simulink model "Project4_MODEL"  (R2023b)
settings: Solver=VariableStepAuto  StartTime=0.0  StopTime=200  RelTol=1e-3
values from neighbouring files (symbols this model uses):
  xp = [sx1 , R*cos(t1) + L , sx2, R*cos(t2)]    [Project_Final_Code.m]
  yp = [sy1, R*sin(t1) + R-offset , sy2 , R*sin(t2) + R-offset]    [Project_Final_Code.m]
undefined symbols (not defined in the file or in its folder): batData, carData, motorData
libraries: slpidlib x1
settings Model: Creator=saman  LastModifiedBy=saman

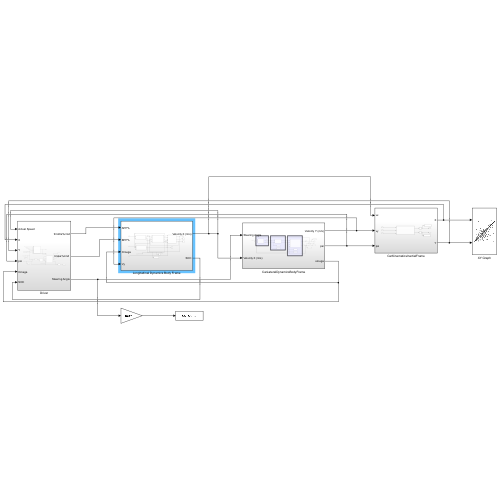
[thumbnail: Simulink's stored preview of the top-level diagram]
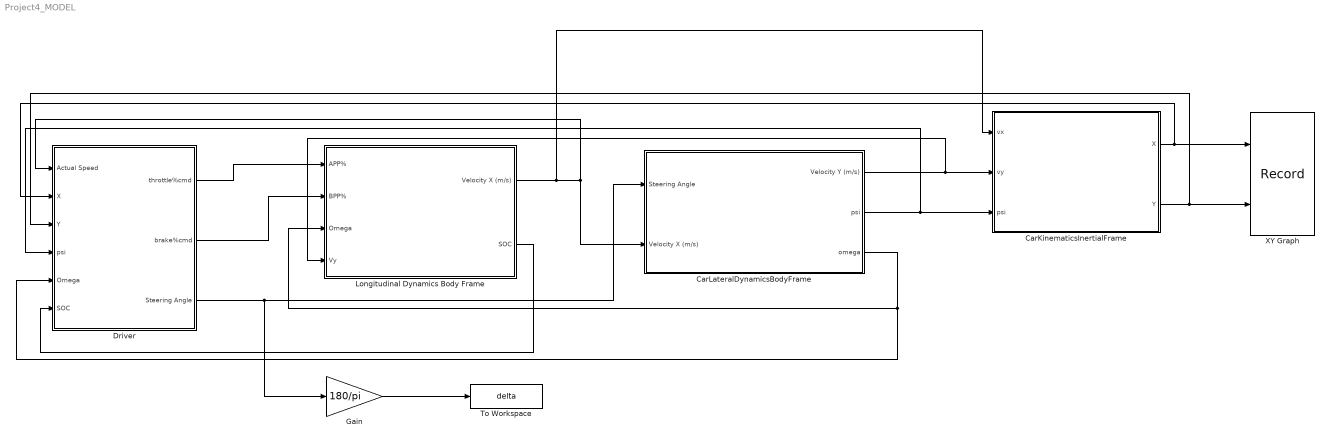
== system Project4_MODEL ==
  CarKinematicsInertialFrame : Subsystem
  CarLateralDynamicsBodyFrame : Subsystem
  "Driver " : Subsystem
  Gain : Gain  Gain=180/pi
  Longitudinal Dynamics Body Frame : Subsystem
  To Workspace : ToWorkspace  VariableName=delta  SaveFormat=Timeseries  SampleTime=-1
  XY Graph : Record  FileSettingsInternal="{\"entries\":[{\"content\":{\"excelSettings\":{\"content\":{},\"type\":\"Streamout.ExcelSettings\"}},\"type\":\"Streamout.FileSettingStorage\",\"uuid\":\"\"}],\"packageUris\":[\"http:\\/\\/schema.mathworks.com\\/mf0\\/streamout_blocks\\/R2020a\"],\"version\":\"1.0\"}"  Layout=[1 1]  SignalsInternal="{\"entries\":[{\"content\":{\"signals\":[{\"content\":{\"blockPath\":[],\"dimensions\":[1],\"domain\":\"\",\"lineColor\":\"#a2142f\",\"plots\":[1],\"port\":1,\"sid\":[\"\"],\"signalID\":55552,\"signalName\":\"CarKinematicsInertialFrame:1\"},\"type\":\"RecordBlkView.Signal\",\"uuid\":\"\"},{\"content\":{\"blockPath\":[],\"dimensions\":[1],\"domain\":\"\",\"lineColor\":\"#139fff\",\"plots\":[1],\"port\":2,\"sid\":[\"\"],\"signalID\":55556,\"signalName\":\"CarKinematicsInertialFrame:2\"},\"type\":\"RecordBlkView.Signal\",\"uuid\":\"\"}]},\"type\":\"RecordBlkView.InputSignals\",\"uuid\":\"\"}],\"packageUris\":[\"http:\\/\\/schema.mathworks.com\\/mf0\\/streamout_blocks\\/R2020a\"],\"version\":\"1.0\"}"  VisualizationBindings="{\"xyplotplugin\":{\"info\":[{\"series\":[{\"bindingParametersList\":[{\"parameter\":\"X-Axis\",\"signalID\":55552,\"signalName\":\"CarKinematicsInertialFrame:1\"},{\"parameter\":\"Y-Axis\",\"signalID\":55556,\"signalName\":\"CarKinematicsInertialFrame:2\"}],\"seriesID\":61892}],\"subplotID\":1}]}}"  CompatibilityTag=XY  st=-1
  wires:
  CarLateralDynamicsBodyFrame/2(psi) -> "Driver "/4(psi), CarKinematicsInertialFrame/3(psi)
  CarKinematicsInertialFrame/2(Y) -> "Driver "/3(Y), XY Graph/2
  CarKinematicsInertialFrame/1(X) -> XY Graph/1, "Driver "/2(X)
  CarLateralDynamicsBodyFrame/1(Velocity Y (m/s)) -> Longitudinal Dynamics Body Frame/4(Vy), CarKinematicsInertialFrame/2(vy)
  "Driver "/1(throttle%cmd) -> Longitudinal Dynamics Body Frame/1(APP%)
  "Driver "/2("brake%cmd ") -> Longitudinal Dynamics Body Frame/2(BPP%)
  Longitudinal Dynamics Body Frame/1(Velocity X (m/s)) -> CarKinematicsInertialFrame/1(vx), "Driver "/1(Actual Speed), CarLateralDynamicsBodyFrame/2(Velocity X (m/s))
  Longitudinal Dynamics Body Frame/2(SOC) -> "Driver "/6(SOC)
  CarLateralDynamicsBodyFrame/3(omega) -> Longitudinal Dynamics Body Frame/3(Omega), "Driver "/5(Omega)
  "Driver "/3(Steering Angle) -> Gain/1, CarLateralDynamicsBodyFrame/1(Steering Angle)
  Gain/1 -> To Workspace/1

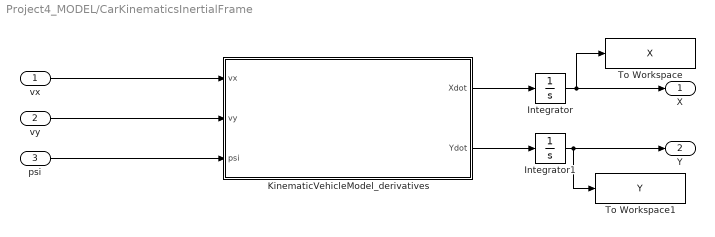
== system Project4_MODEL/CarKinematicsInertialFrame ==
  vx : Inport
  vy : Inport  Port=2
  psi : Inport  Port=3
  Integrator : Integrator  InitialCondition=carData.init.X0
  Integrator1 : Integrator  InitialCondition=carData.init.Y0
  KinematicVehicleModel_derivatives : MATLAB Function  TreatAsAtomicUnit=on  mask{obj=carData}
      mask prompts: obj "obj structure"
  To Workspace : ToWorkspace  VariableName=X  SaveFormat=Timeseries  SampleTime=-1
  To Workspace1 : ToWorkspace  VariableName=Y  SaveFormat=Timeseries  SampleTime=-1
  X : Outport
  Y : Outport  Port=2
  wires:
  KinematicVehicleModel_derivatives/1(Xdot) -> Integrator/1
  KinematicVehicleModel_derivatives/2(Ydot) -> Integrator1/1
  Integrator/1 -> To Workspace/1, X/1
  Integrator1/1 -> To Workspace1/1, Y/1
  vx/1 -> KinematicVehicleModel_derivatives/1(vx)
  vy/1 -> KinematicVehicleModel_derivatives/2(vy)
  psi/1 -> KinematicVehicleModel_derivatives/3(psi)

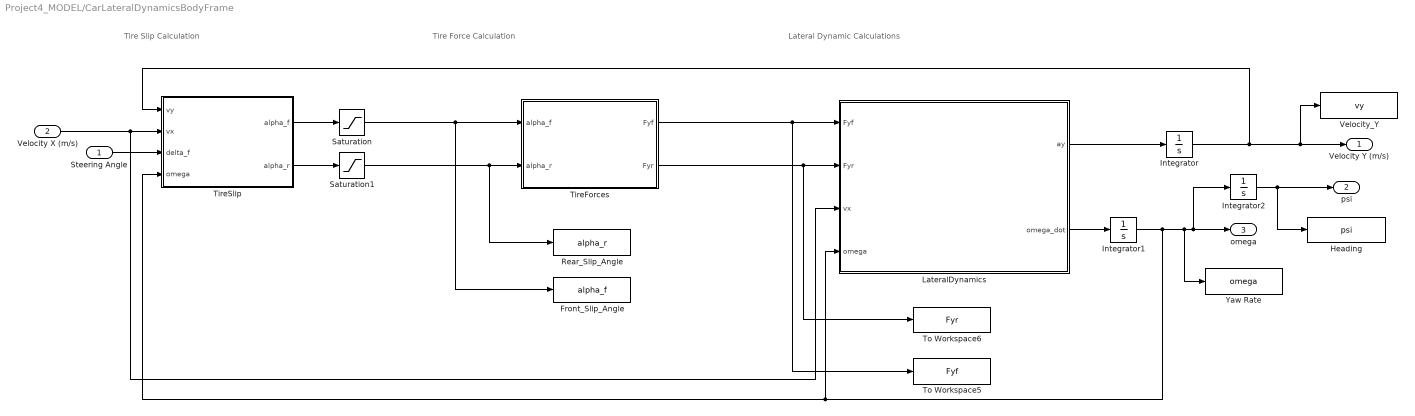
== system Project4_MODEL/CarLateralDynamicsBodyFrame ==
  note: Tire Slip Calculation
  note: Tire Force Calculation
  note: Lateral Dynamic Calculations
  Steering Angle : Inport
  Velocity X (m/s) : Inport  Port=2
  Front_Slip_Angle : ToWorkspace  VariableName=alpha_f  SaveFormat=Timeseries  SampleTime=-1
  Heading : ToWorkspace  VariableName=psi  SaveFormat=Timeseries  SampleTime=-1
  Integrator : Integrator  InitialCondition=carData.init.vy0
  Integrator1 : Integrator  InitialCondition=carData.init.omega0
  Integrator2 : Integrator  InitialCondition=carData.init.psi0
  LateralDynamics : MATLAB Function  TreatAsAtomicUnit=on  mask{obj=carData}
      mask prompts: obj "obj structure"
  Rear_Slip_Angle : ToWorkspace  VariableName=alpha_r  SaveFormat=Timeseries  SampleTime=-1
  Saturation : Saturate  UpperLimit=carData.maxAlpha  LowerLimit=-carData.maxAlpha
  Saturation1 : Saturate  UpperLimit=carData.maxAlpha  LowerLimit=-carData.maxAlpha
  TireForces : MATLAB Function  TreatAsAtomicUnit=on  mask{obj=carData}
      mask prompts: obj "obj structure"
  TireSlip : MATLAB Function  TreatAsAtomicUnit=on  mask{obj=carData}
      mask prompts: obj "obj structure"
  To Workspace5 : ToWorkspace  VariableName=Fyf  SaveFormat=Timeseries  SampleTime=-1
  To Workspace6 : ToWorkspace  VariableName=Fyr  SaveFormat=Timeseries  SampleTime=-1
  Velocity_Y : ToWorkspace  VariableName=vy  SaveFormat=Timeseries  SampleTime=-1
  Yaw Rate : ToWorkspace  VariableName=omega  SaveFormat=Timeseries  SampleTime=-1
  Velocity Y (m/s) : Outport
  psi : Outport  Port=2
  omega : Outport  Port=3
  wires:
  LateralDynamics/1(ay) -> Integrator/1
  Integrator/1 -> Velocity Y (m/s)/1, Velocity_Y/1, TireSlip/1(vy)
  LateralDynamics/2(omega_dot) -> Integrator1/1
  Integrator1/1 -> Integrator2/1, omega/1, Yaw Rate/1, LateralDynamics/4(omega), TireSlip/4(omega)
  TireSlip/1(alpha_f) -> Saturation/1
  TireSlip/2(alpha_r) -> Saturation1/1
  TireForces/1(Fyf) -> LateralDynamics/1(Fyf), To Workspace5/1
  TireForces/2(Fyr) -> LateralDynamics/2(Fyr), To Workspace6/1
  Saturation/1 -> TireForces/1(alpha_f), Front_Slip_Angle/1
  Saturation1/1 -> TireForces/2(alpha_r), Rear_Slip_Angle/1
  Velocity X (m/s)/1 -> TireSlip/2(vx), LateralDynamics/3(vx)
  Steering Angle/1 -> TireSlip/3(delta_f)
  Integrator2/1 -> Heading/1, psi/1

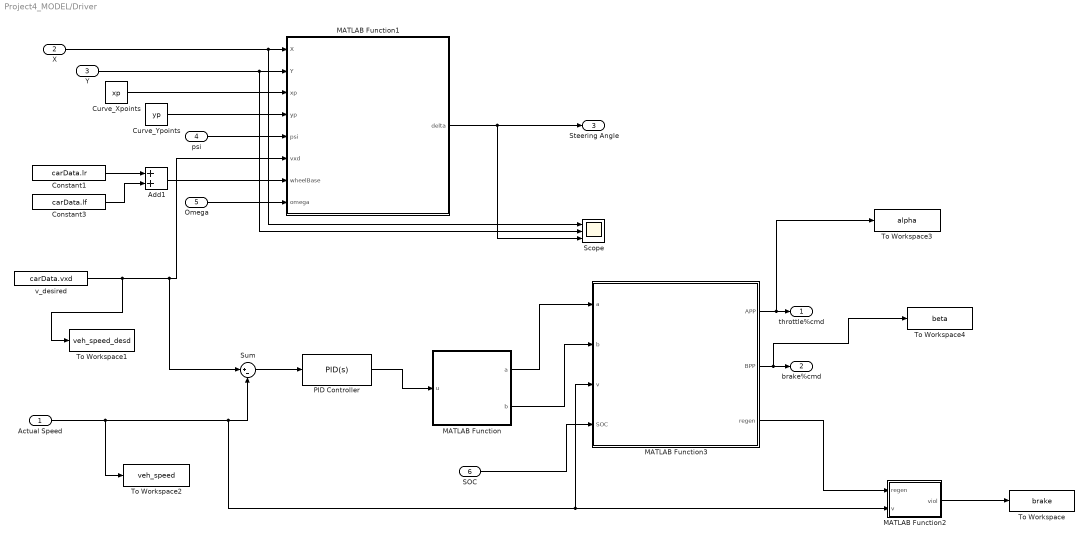
== system Project4_MODEL/Driver  ==
  Actual Speed : Inport
  X : Inport  Port=2
  Y : Inport  Port=3
  psi : Inport  Port=4
  Omega : Inport  Port=5
  SOC : Inport  Port=6
  Add1 : Sum
  Constant1 : Constant  Value=carData.lr
  Constant3 : Constant  Value=carData.lf
  Curve_Xpoints : Constant  Value=xp  VectorParams1D=off
  Curve_Ypoints : Constant  Value=yp  VectorParams1D=off
  MATLAB Function : MATLAB Function  TreatAsAtomicUnit=on
  MATLAB Function1 : MATLAB Function  TreatAsAtomicUnit=on
  MATLAB Function2 : MATLAB Function  TreatAsAtomicUnit=on
  MATLAB Function3 : MATLAB Function  TreatAsAtomicUnit=on
  PID Controller : slpidlib/PID Controller  Controller=PID  Form=Parallel  TimeDomain=Continuous-time  UseExternalTs=off  SampleTime=-1  IntegratorMethod=Forward Euler  FilterMethod=Forward Euler  ControllerParametersSource=internal  P=2.5  I=.1  UseKiTs=off  D=.5  N=100  UseFilter=on  TunerSelectOption=Transfer Function Based (PID Tuner App)  InitialConditionSource=internal  InitialConditionForIntegrator=0  InitialConditionForFilter=0  DifferentiatorICPrevScaledInput=0  ExternalReset=none  TrackingMode=off  Kt=1  LimitOutput=on  SatLimitsSource=internal  UpperSaturationLimit=1  LowerSaturationLimit=-1  LinearizeAsGain=off  AntiWindupMode=none  Kb=1  LimitIntegrator=off  UpperIntegratorSaturationLimit=inf  LowerIntegratorSaturationLimit=-inf  POutMin=[]  POutMax=[]  IOutMin=[]  IOutMax=[]  DOutMin=[]  DOutMax=[]  NOutMin=[]  NOutMax=[]  SumOutMin=[]  SumOutMax=[]  SaturationOutMin=[]  SaturationOutMax=[]  PParamMin=[]  PParamMax=[]  IParamMin=[]  IParamMax=[]  DParamMin=[]  DParamMax=[]  NParamMin=[]  NParamMax=[]  KbParamMin=[]  KbParamMax=[]  KtParamMin=[]  KtParamMax=[]  KbOutMin=[]  KbOutMax=[]  KtOutMin=[]  KtOutMax=[]  IntegratorOutMin=[]  IntegratorOutMax=[]  FilterOutMin=[]  FilterOutMax=[]  SumI1OutMin=[]  SumI1OutMax=[]  SumI2OutMin=[]  SumI2OutMax=[]  SumI3OutMin=[]  SumI3OutMax=[]  SumI4OutMin=[]  SumI4OutMax=[]  SumDOutMin=[]  SumDOutMax=[]  DifferentiatorOutMin=[]  DifferentiatorOutMax=[]  FilterDiffOutCoefMin=[]  FilterDiffOutCoefMax=[]  ReciprocalOutMin=[]  ReciprocalOutMax=[]  SumDenOutMin=[]  SumDenOutMax=[]  SumNumOutMin=[]  SumNumOutMax=[]  DivideOutMin=[]  DivideOutMax=[]  UdiffTsProdOutMin=[]  UdiffTsProdOutMax=[]  NTsProdOutMin=[]  NTsProdOutMax=[]  UintegralTsProdOutMin=[]  UintegralTsProdOutMax=[]  UngainTsProdOutMin=[]  UngainTsProdOutMax=[]  ClampingZeroOutDataTypeStr=Inherit: Inherit via back propagation  ClampingZeroOutMin=[]  ClampingZeroOutMax=[]  FilterDenConstantOutDataTypeStr=Inherit: Inherit via back propagation  FilterDenConstantOutMin=[]  FilterDenConstantOutMax=[]  PCopyOutDataTypeStr=Inherit: Inherit via back propagation  PCopyOutMin=[]  PCopyOutMax=[]  NCopyOutDataTypeStr=Inherit: Inherit via back propagation  NCopyOutMin=[]  NCopyOutMax=[]  IntegratorContinuousStateAttributes=''  IntegratorStateMustResolveToSignalObject=off  IntegratorRTWStateStorageClass=Auto  FilterContinuousStateAttributes=''  FilterStateMustResolveToSignalObject=off  FilterRTWStateStorageClass=Auto  ParallelPVariant=InternalParameters  IdealPVariant=Disabled  IVariant=InternalParameters  DVariant=InternalParameters  IntegratorVariant=Continuous  SatVariant=Enabled  AWVariant=Passthrough  PCopyVariant=Disabled  TRVariant=Disabled  FdbkBlocksVariant=Forward  IdealPFdbkVariant=Disabled  SatFdbkVariant=Disabled  DerivativeFilterVariant=ContFilter  NVariant=InternalParameters  NCopyVariant=Disabled  FilterICVariant=InternalICsFilter  IntegratorICVariant=InternalICs  ExternalResetVariant=Disabled  TRSumVariant=Passthrough  SumFdbkVariant=Disabled  SumVariant=Sum_PID  TsampFilterVariant=InternalTs  TsampNgainVariant=Passthrough  TsampIntegralVariant=Disabled_SignalSpec  ExternalSaturationOutDataTypeStr=Inherit: Same as second input
  Scope : Scope  NumInputPorts=3
  Sum : Sum  Inputs=|+-
  To Workspace : ToWorkspace  VariableName=brake  SaveFormat=Timeseries  SampleTime=-1
  To Workspace1 : ToWorkspace  VariableName=veh_speed_desd  SaveFormat=Timeseries  SampleTime=-1
  To Workspace2 : ToWorkspace  VariableName=veh_speed  SaveFormat=Timeseries  SampleTime=-1
  To Workspace3 : ToWorkspace  VariableName=alpha  SaveFormat=Timeseries  SampleTime=-1
  To Workspace4 : ToWorkspace  VariableName=beta  SaveFormat=Timeseries  SampleTime=-1
  v_desired : Constant  Value=carData.vxd
  throttle%cmd : Outport
  "brake%cmd " : Outport  Port=2
  Steering Angle : Outport  Port=3
  wires:
  v_desired/1 -> To Workspace1/1, Sum/1, MATLAB Function1/6(vxd)
  Actual Speed/1 -> To Workspace2/1, MATLAB Function3/3(v), MATLAB Function2/2(v), Sum/2
  Sum/1 -> PID Controller/1
  PID Controller/1 -> MATLAB Function/1(u)
  Omega/1 -> MATLAB Function1/8(omega)
  Curve_Ypoints/1 -> MATLAB Function1/4(yp)
  psi/1 -> MATLAB Function1/5(psi)
  X/1 -> Scope/1, MATLAB Function1/1(X)
  Curve_Xpoints/1 -> MATLAB Function1/3(xp)
  MATLAB Function1/1(delta) -> Steering Angle/1, Scope/3
  Y/1 -> Scope/2, MATLAB Function1/2(Y)
  Constant3/1 -> Add1/2
  Constant1/1 -> Add1/1
  Add1/1 -> MATLAB Function1/7(wheelBase)
  MATLAB Function/1(a) -> MATLAB Function3/1(a)
  MATLAB Function/2(b) -> MATLAB Function3/2(b)
  MATLAB Function2/1(viol) -> To Workspace/1
  SOC/1 -> MATLAB Function3/4(SOC)
  MATLAB Function3/3(regen) -> MATLAB Function2/1(regen)
  MATLAB Function3/2(BPP) -> To Workspace4/1, "brake%cmd "/1
  MATLAB Function3/1(APP) -> To Workspace3/1, throttle%cmd/1

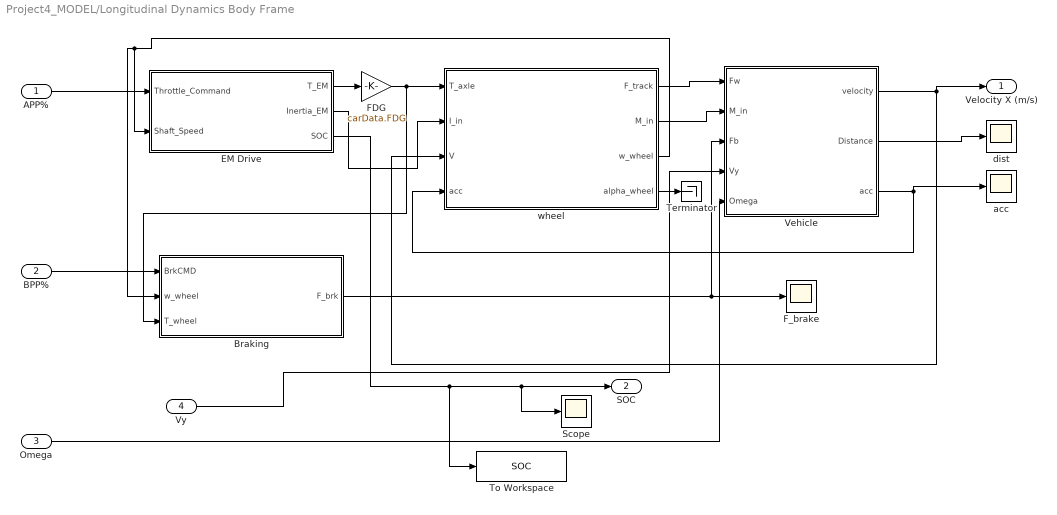
== system Project4_MODEL/Longitudinal Dynamics Body Frame ==
  APP% : Inport
  BPP% : Inport  Port=2
  Omega : Inport  Port=3
  Vy : Inport  Port=4
  Braking : Subsystem
  EM Drive : Subsystem
  FDG : Gain  Gain=carData.FDG
  F_brake : Scope
  Scope : Scope
  Terminator : Terminator
  To Workspace : ToWorkspace  VariableName=SOC  SaveFormat=Timeseries  SampleTime=-1
  Vehicle : Subsystem
  acc : Scope
  dist : Scope
  "wheel " : Subsystem
  Velocity X (m/s) : Outport
  SOC : Outport  Port=2
  wires:
  "wheel "/3(w_wheel) -> Braking/2("w_wheel "), EM Drive/2(Shaft_Speed)
  Vehicle/3(acc) -> acc/1, "wheel "/4(acc)
  Braking/1("F_brk ") -> Vehicle/3("Fb "), F_brake/1
  "wheel "/2(M_in) -> Vehicle/2("M_in ")
  Vehicle/1("velocity ") -> Velocity X (m/s)/1, "wheel "/3(V)
  "wheel "/1(F_track) -> Vehicle/1("Fw ")
  EM Drive/3(SOC) -> To Workspace/1, Scope/1, SOC/1
  FDG/1 -> Braking/3(T_wheel), "wheel "/1(T_axle)
  EM Drive/2(Inertia_EM) -> "wheel "/2(I_in)
  Vehicle/2("Distance ") -> dist/1
  "wheel "/4(alpha_wheel) -> Terminator/1
  EM Drive/1(T_EM) -> FDG/1
  APP%/1 -> EM Drive/1(Throttle_Command)
  BPP%/1 -> Braking/1("BrkCMD ")
  Vy/1 -> Vehicle/4(Vy)
  Omega/1 -> Vehicle/5(Omega)

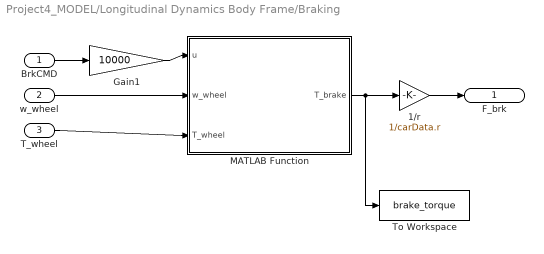
== system Project4_MODEL/Longitudinal Dynamics Body Frame/Braking ==
  "BrkCMD " : Inport
  "w_wheel " : Inport  Port=2
  T_wheel : Inport  Port=3
  1/r : Gain  Gain=1/carData.r
  Gain1 : Gain  Gain=10000
  MATLAB Function : MATLAB Function  TreatAsAtomicUnit=on
  To Workspace : ToWorkspace  VariableName=brake_torque  SaveFormat=Timeseries  SampleTime=-1
  "F_brk " : Outport  VectorParamsAs1DForOutWhenUnconnected=off
  wires:
  "BrkCMD "/1 -> Gain1/1
  Gain1/1 -> MATLAB Function/1(u)
  MATLAB Function/1(T_brake) -> To Workspace/1, 1/r/1
  "w_wheel "/1 -> MATLAB Function/2(w_wheel)
  T_wheel/1 -> MATLAB Function/3(T_wheel)
  1/r/1 -> "F_brk "/1

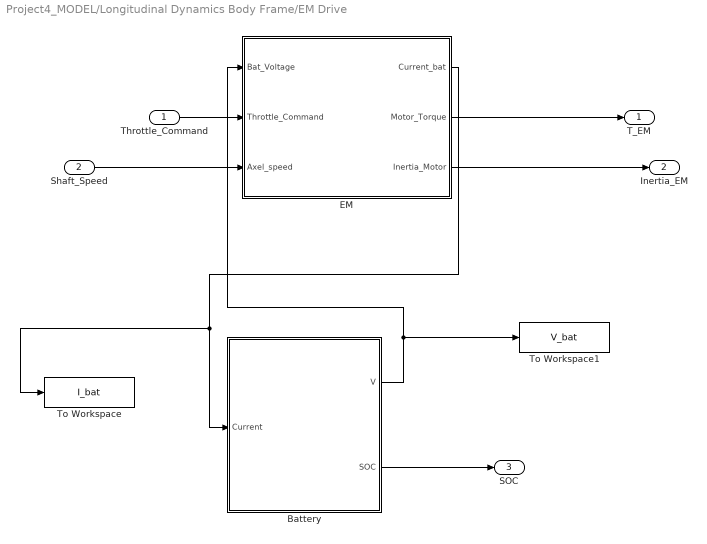
== system Project4_MODEL/Longitudinal Dynamics Body Frame/EM Drive ==
  Throttle_Command : Inport
  Shaft_Speed : Inport  Port=2
  Battery : Subsystem
  EM : Subsystem
  To Workspace : ToWorkspace  VariableName=I_bat  SaveFormat=Timeseries  SampleTime=-1
  To Workspace1 : ToWorkspace  VariableName=V_bat  SaveFormat=Timeseries  SampleTime=-1
  T_EM : Outport
  Inertia_EM : Outport  Port=2
  SOC : Outport  Port=3
  wires:
  EM/1(Current_bat) -> To Workspace/1, Battery/1(Current)
  Throttle_Command/1 -> EM/2(Throttle_Command)
  Shaft_Speed/1 -> EM/3(Axel_speed)
  EM/2(Motor_Torque) -> T_EM/1
  EM/3(Inertia_Motor) -> Inertia_EM/1
  Battery/1(V) -> To Workspace1/1, EM/1(Bat_Voltage)
  Battery/2(SOC) -> SOC/1

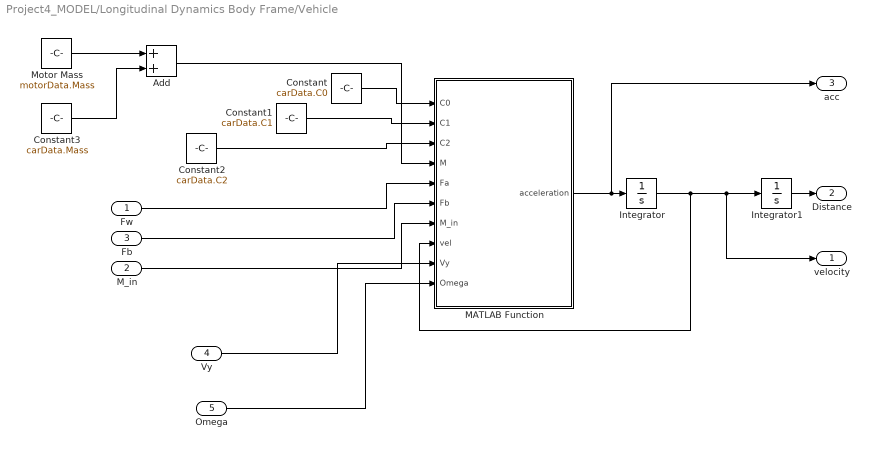
== system Project4_MODEL/Longitudinal Dynamics Body Frame/Vehicle ==
  "Fw " : Inport
  "M_in " : Inport  Port=2
  "Fb " : Inport  Port=3
  Vy : Inport  Port=4
  Omega : Inport  Port=5
  Add : Sum
  Constant : Constant  Value=carData.C0
  Constant1 : Constant  Value=carData.C1
  Constant2 : Constant  Value=carData.C2
  Constant3 : Constant  Value=carData.Mass
  Integrator : Integrator  LimitOutput=on  LowerSaturationLimit=0
  Integrator1 : Integrator
  MATLAB Function : MATLAB Function  TreatAsAtomicUnit=on
  Motor Mass : Constant  Value=motorData.Mass
  "velocity " : Outport  VectorParamsAs1DForOutWhenUnconnected=off
  "Distance " : Outport  Port=2  VectorParamsAs1DForOutWhenUnconnected=off
  acc : Outport  Port=3
  wires:
  Constant1/1 -> MATLAB Function/2(C1)
  Constant/1 -> MATLAB Function/1(C0)
  MATLAB Function/1(acceleration) -> acc/1, Integrator/1
  Constant2/1 -> MATLAB Function/3(C2)
  Constant3/1 -> Add/2
  "Fw "/1 -> MATLAB Function/5(Fa)
  "Fb "/1 -> MATLAB Function/6(Fb)
  Integrator/1 -> MATLAB Function/8(vel), "velocity "/1, Integrator1/1
  Integrator1/1 -> "Distance "/1
  "M_in "/1 -> MATLAB Function/7(M_in)
  Motor Mass/1 -> Add/1
  Add/1 -> MATLAB Function/4(M)
  Vy/1 -> MATLAB Function/9(Vy)
  Omega/1 -> MATLAB Function/10(Omega)

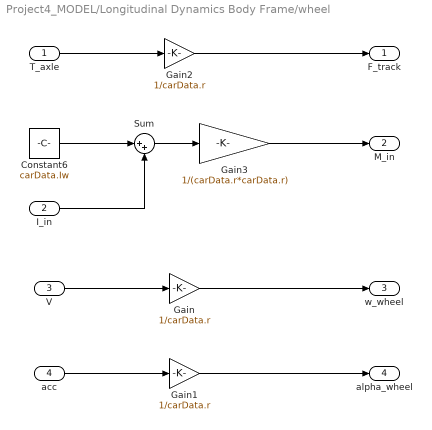
== system Project4_MODEL/Longitudinal Dynamics Body Frame/wheel  ==
  T_axle : Inport
  I_in : Inport  Port=2
  V : Inport  Port=3
  acc : Inport  Port=4
  Constant6 : Constant  Value=carData.Iw
  Gain : Gain  Gain=1/carData.r
  Gain1 : Gain  Gain=1/carData.r
  Gain2 : Gain  Gain=1/carData.r
  Gain3 : Gain  Gain=1/(carData.r*carData.r)
  Sum : Sum  Inputs=|++
  F_track : Outport
  M_in : Outport  Port=2
  w_wheel : Outport  Port=3
  alpha_wheel : Outport  Port=4
  wires:
  Gain/1 -> w_wheel/1
  V/1 -> Gain/1
  acc/1 -> Gain1/1
  Gain1/1 -> alpha_wheel/1
  T_axle/1 -> Gain2/1
  Gain2/1 -> F_track/1
  Gain3/1 -> M_in/1
  Constant6/1 -> Sum/1
  I_in/1 -> Sum/2
  Sum/1 -> Gain3/1

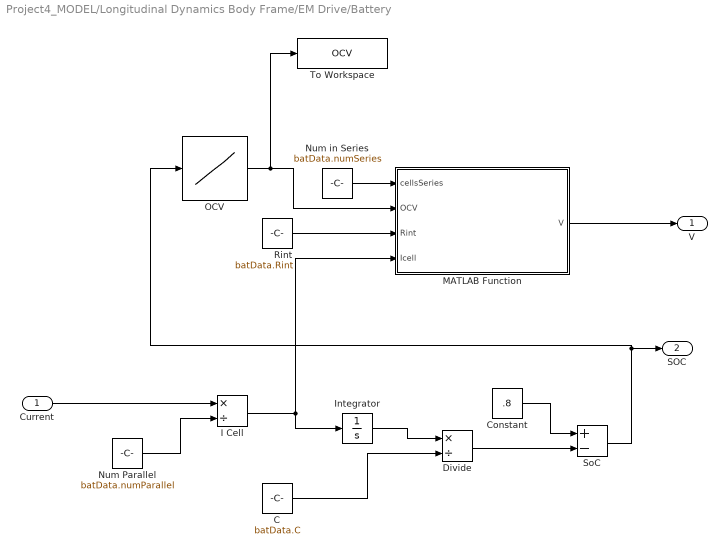
== system Project4_MODEL/Longitudinal Dynamics Body Frame/EM Drive/Battery ==
  Current : Inport
  C : Constant  Value=batData.C
  Constant : Constant  Value=.8
  Divide : Product  Inputs=*/
  I Cell : Product  Inputs=*/
  Integrator : Integrator
  MATLAB Function : MATLAB Function  TreatAsAtomicUnit=on
  Num Parallel : Constant  Value=batData.numParallel
  Num in Series : Constant  Value=batData.numSeries
  OCV : Lookup_n-D  NumberOfTableDimensions=1  BreakpointsForDimension1=batData.SOC  BreakpointsForDimension2=[1:3]  Table=batData.OCV  InternalRulePriority=Speed  RndMeth=Simplest
  Rint : Constant  Value=batData.Rint
  SoC : Sum  Inputs=+-
  To Workspace : ToWorkspace  VariableName=OCV  SaveFormat=Timeseries  SampleTime=-1
  V : Outport
  SOC : Outport  Port=2
  wires:
  Num Parallel/1 -> I Cell/2
  I Cell/1 -> Integrator/1, MATLAB Function/4(Icell)
  C/1 -> Divide/2
  Integrator/1 -> Divide/1
  Divide/1 -> SoC/2
  SoC/1 -> SOC/1, OCV/1
  MATLAB Function/1(V) -> V/1
  OCV/1 -> To Workspace/1, MATLAB Function/2(OCV)
  Rint/1 -> MATLAB Function/3(Rint)
  Num in Series/1 -> MATLAB Function/1(cellsSeries)
  Constant/1 -> SoC/1
  Current/1 -> I Cell/1

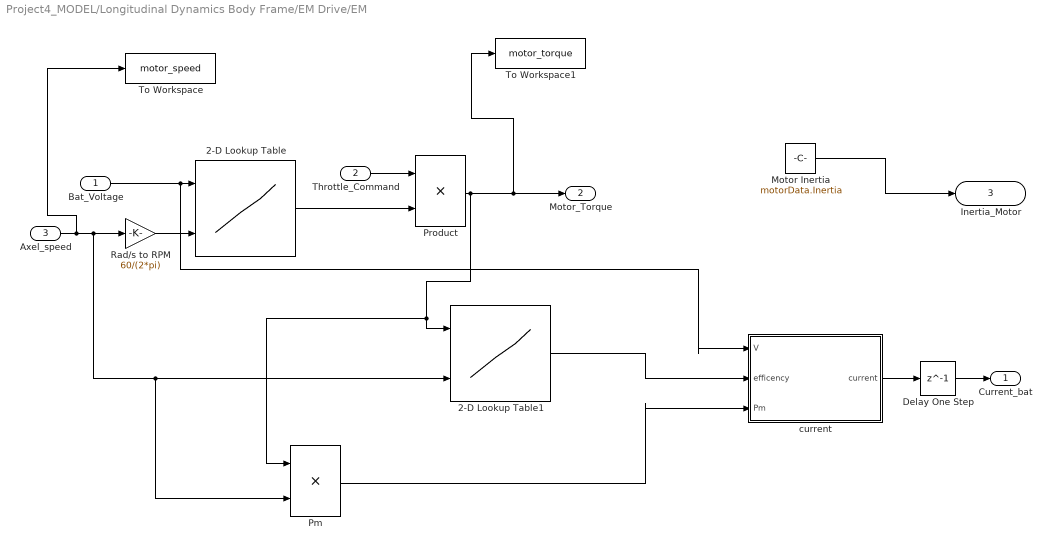
== system Project4_MODEL/Longitudinal Dynamics Body Frame/EM Drive/EM ==
  Bat_Voltage : Inport
  Throttle_Command : Inport  Port=2
  Axel_speed : Inport  Port=3
  2-D Lookup Table : Lookup_n-D  BreakpointsForDimension1=motorData.vbus  BreakpointsForDimension2=motorData.rpm  Table=motorData.maxtorque  InternalRulePriority=Speed  RndMeth=Simplest
      settings: InputPortMap=u0,u1
  2-D Lookup Table1 : Lookup_n-D  BreakpointsForDimension1=motorData.eta_torque  BreakpointsForDimension2=motorData.eta_speed  Table=motorData.eta_val  InternalRulePriority=Speed  RndMeth=Simplest
      settings: InputPortMap=u0,u1
  Delay One Step : Delay  DelayLength=1
  Motor Inertia : Constant  Value=motorData.Inertia
  Pm : Product
  Product : Product
  Rad/s to RPM : Gain  Gain=60/(2*pi)
  To Workspace : ToWorkspace  VariableName=motor_speed  SaveFormat=Timeseries  SampleTime=-1
  To Workspace1 : ToWorkspace  VariableName=motor_torque  SaveFormat=Timeseries  SampleTime=-1
  current : MATLAB Function  TreatAsAtomicUnit=on
  Current_bat : Outport
  Motor_Torque : Outport  Port=2
  Inertia_Motor : Outport  Port=3
  wires:
  Axel_speed/1 -> To Workspace/1, Rad/s to RPM/1, 2-D Lookup Table1/2, Pm/2
  Bat_Voltage/1 -> current/1(V), 2-D Lookup Table/1
  2-D Lookup Table/1 -> Product/2
  Throttle_Command/1 -> Product/1
  Product/1 -> Pm/1, 2-D Lookup Table1/1, To Workspace1/1, Motor_Torque/1
  Pm/1 -> current/3(Pm)
  2-D Lookup Table1/1 -> current/2(efficency)
  Motor Inertia/1 -> Inertia_Motor/1
  current/1(current) -> Delay One Step/1
  Rad/s to RPM/1 -> 2-D Lookup Table/2
  Delay One Step/1 -> Current_bat/1

== matlab function Project4_MODEL/CarLateralDynamicsBodyFrame/TireSlip ==
  data: vy input size=1; vx input; delta_f input size=1; omega input; alpha_f output; obj parameter; alpha_r output
function [alpha_f, alpha_r] = fcn(vy,  vx, delta_f, omega, obj)

if abs(vx)> obj.vx_threshold1
      alpha_f = delta_f - (vy + omega * obj.lf) / vx;
      alpha_r = - (vy - omega * obj.lr) / vx;
else
      alpha_f = 0;
      alpha_r = 0;
end
end
% if abs(vx)> obj.vx_threshold1
%       alpha_f = delta_f - atan2(vy + omega * obj.lf,vx);
%       alpha_r = atan2(vy - omega * obj.lr,vx);
% else
%       alpha_f = 0;
%       alpha_r = 0;
% end
% end

== matlab function Project4_MODEL/Driver /MATLAB Function2 ==
  data: regen input; viol output; v input
function viol = fcn(regen, v)

    speed = (3600/1600)*v;
    if speed < 5
        regen_vio = 0;
        if regen == regen_vio
            viol = 0;
        else
            viol = 0;

        end
    elseif speed== 25
        regen_vio = 0.95;
        if regen == regen_vio
            viol = 0;
        else
            viol = 0;
        end
    elseif v > 25
        regen_vio = 0.95;
        if regen == regen_vio
            viol = 0;
        else 
            viol = 0;
        end
    else
        regen_vio = ((0.95/20)*speed) - 0.2375;
        if regen == regen_vio
            viol=0;
        else
            viol = 0;
        end
    end

== matlab function Project4_MODEL/Driver /MATLAB Function1 ==
  data: X input; delta output; Y input; xp input; yp input; psi input; vxd input; wheelBase input; omega input
function delta = SimplestDriver(X,Y,xp,yp,psi,vxd,wheelBase,omega)

%Find closest point on curve to car location
point = [X,Y];
distance = [];
curve = [xp;yp];
for i = 1:length(curve)
     distance(end+1) = ((curve(1,i)-point(1))^2+(curve(2,i)-point(2))^2)^(1/2);
end
[~,min_index] = min(distance);
k = min_index +10; %Going two point up the curve for a smoother turn
%To prevent out of bounds index
if(k>length(curve))
    k = length(curve);
end
target_point = curve(:,k);

alpha = atan2(target_point(2)-point(2), target_point(1)-point(1))-psi;
psi_dot = 2*vxd*sin(alpha)/wheelBase;
delta = psi_dot-omega;
% delta = atan2(2*wheelBase*sin(alpha),1);
%delta = atan2(2*wheelBase*sin(alpha),10);
% delta = 0;
% if X>900
%     delta = 5;
% end

== matlab function Project4_MODEL/Driver /MATLAB Function3 ==
  data: a input; APP output; b input; v input; SOC input; BPP output; regen output
function [APP, BPP, regen] = fcn(a,b,v, SOC)

if a >= 0
    APP = a;
    regen  = 0;
    BPP = 0;
else
    APP = 0.1*b;
    BPP = 0.9*b;
    regen = APP;
end

== matlab function Project4_MODEL/Driver /MATLAB Function ==
  data: u input; a output; b output
function [a,b] = fcn(u)

if u>0
    acc=u;
    brk=0;
elseif u<0
    acc=0;
    brk=u;
else
    acc=0;
    brk=0;
end
a= acc;
b= brk;

== matlab function Project4_MODEL/Longitudinal Dynamics Body Frame/Vehicle/MATLAB Function ==
  data: C0 input; acceleration output; C1 input; C2 input; M input; Fa input; Fb input; M_in input; vel input; Vy input; Omega input
function acceleration   = vehicle(C0,C1,C2,M,Fa,Fb,M_in, vel, Vy, Omega)

acceleration = (((Fa-Fb))-(C0+ C1*vel + C2*(vel)^2))/(M+M_in)+ (Vy*Omega);

== matlab function Project4_MODEL/Longitudinal Dynamics Body Frame/EM Drive/EM/current ==
  data: V input; current output; efficency input; Pm input
function current = fcn(V,efficency,Pm)

current = (Pm*efficency^(Pm/(abs(Pm)+.001)))/V;

== matlab function Project4_MODEL/Longitudinal Dynamics Body Frame/EM Drive/Battery/MATLAB Function ==
  data: cellsSeries input; V output; OCV input; Rint input; Icell input
function V = fcn(cellsSeries,OCV,Rint,Icell)

V = cellsSeries*(OCV-Rint*Icell);

== matlab function Project4_MODEL/CarKinematicsInertialFrame/KinematicVehicleModel_derivatives ==
  data: vx input; vy input; psi input size=1; Xdot output; Ydot output
function [Xdot, Ydot] = fcn(vx, vy, psi)
    temp = TF(psi) * [vx;vy]; 
    Xdot = temp(1);
    Ydot = temp(2);
  
end

function y = TF(psi)
    y = [cos(psi), -sin(psi); sin(psi), cos(psi)];
end

== matlab function Project4_MODEL/CarLateralDynamicsBodyFrame/LateralDynamics ==
  data: Fyf input; Fyr input size=1; vx input; omega input; ay output; obj parameter; omega_dot output
function [ay, omega_dot] = fcn(Fyf, Fyr, vx, omega, obj)

Fy = Fyf + Fyr;
ay = Fy / obj.Mass - omega * vx;
        
M  = Fyf * obj.lf - Fyr * obj.lr;        
omega_dot = M / obj.Inertia;        

end

== matlab function Project4_MODEL/Longitudinal Dynamics Body Frame/Braking/MATLAB Function ==
  data: u input; T_brake output; w_wheel input; T_wheel input
function T_brake = fcn(u,w_wheel,T_wheel)
%y = u*sign(w_wheel);
%y = 4*u * v/(abs(v)+0.0001);
%y = u;
Tb_cap = -u;
if w_wheel == 0
    T_brake = min(abs(T_wheel),Tb_cap)*w_wheel/(abs(w_wheel+.0001));
else
    T_brake =Tb_cap*w_wheel/(abs(w_wheel+.0001));
end

== matlab function Project4_MODEL/CarLateralDynamicsBodyFrame/TireForces ==
  data: alpha_f input; alpha_r input; Fyf output; obj parameter; Fyr output
function [Fyf, Fyr] = fcn(alpha_f, alpha_r, obj)

Fyf = min(obj.Fyfmax,obj.Calpha_f * alpha_f);
Fyr = min(obj.Fyrmax, obj.Calpha_r * alpha_r);
end
